simulink model "zeroovershoot"  (R2023a)
settings: Solver=VariableStepAuto  StartTime=0.0  StopTime=30  RelTol=1e-3
model workspace (MAT data in the model file):
  lambda = 0.98
libraries: slpidlib x2, cstblocks x1
settings Model: Creator=ritwi  LastModifiedBy=ritwi

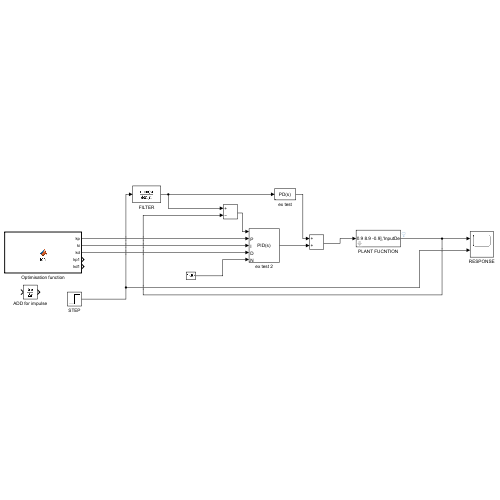
[thumbnail: Simulink's stored preview of the top-level diagram]
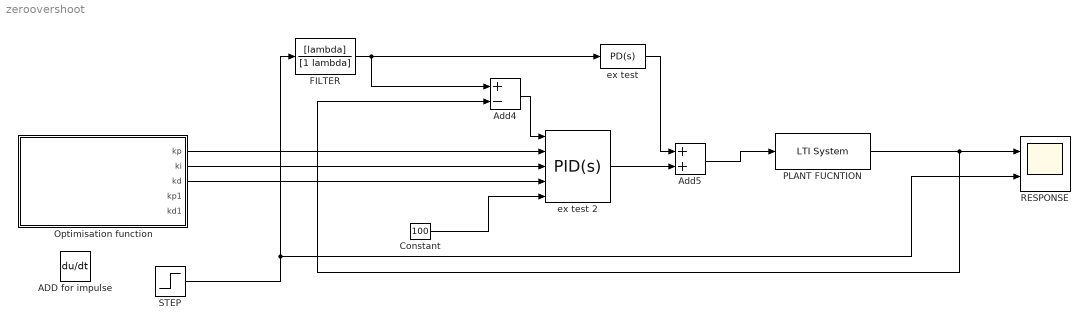
== system zeroovershoot ==
  ADD for impulse : Derivative
  Add4 : Sum  Inputs=+-
  Add5 : Sum
  Constant : Constant  Value=100
  FILTER : TransferFcn  Numerator=[lambda]  Denominator=[1 lambda]
  Optimisation function : MATLAB Function  TreatAsAtomicUnit=on
  PLANT FUCNTION : cstblocks/LTI System  sys=tf([1 ],[1 0.9 8.9 -0.9],'InputDelay',0.2)  IC=[]
  RESPONSE : Scope  NumInputPorts=2
  STEP : Step  After=1000  SampleTime=0
  ex test : slpidlib/PID Controller  Controller=PD  Form=Parallel  TimeDomain=Continuous-time  UseExternalTs=off  SampleTime=-1  IntegratorMethod=Forward Euler  FilterMethod=Forward Euler  ControllerParametersSource=internal  P=-1.2562  I=0  UseKiTs=off  D=7.6042  N=1000  UseFilter=on  TunerSelectOption=Transfer Function Based (PID Tuner App)  InitialConditionSource=internal  InitialConditionForIntegrator=0  InitialConditionForFilter=0  DifferentiatorICPrevScaledInput=0  ExternalReset=none  TrackingMode=off  Kt=1  LimitOutput=off  SatLimitsSource=internal  UpperSaturationLimit=inf  LowerSaturationLimit=-inf  LinearizeAsGain=on  AntiWindupMode=none  Kb=1  LimitIntegrator=off  UpperIntegratorSaturationLimit=inf  LowerIntegratorSaturationLimit=-inf  POutMin=[]  POutMax=[]  IOutMin=[]  IOutMax=[]  DOutMin=[]  DOutMax=[]  NOutMin=[]  NOutMax=[]  SumOutMin=[]  SumOutMax=[]  SaturationOutMin=[]  SaturationOutMax=[]  PParamMin=[]  PParamMax=[]  IParamMin=[]  IParamMax=[]  DParamMin=[]  DParamMax=[]  NParamMin=[]  NParamMax=[]  KbParamMin=[]  KbParamMax=[]  KtParamMin=[]  KtParamMax=[]  KbOutMin=[]  KbOutMax=[]  KtOutMin=[]  KtOutMax=[]  IntegratorOutMin=[]  IntegratorOutMax=[]  FilterOutMin=[]  FilterOutMax=[]  SumI1OutMin=[]  SumI1OutMax=[]  SumI2OutMin=[]  SumI2OutMax=[]  SumI3OutMin=[]  SumI3OutMax=[]  SumI4OutMin=[]  SumI4OutMax=[]  SumDOutMin=[]  SumDOutMax=[]  DifferentiatorOutMin=[]  DifferentiatorOutMax=[]  FilterDiffOutCoefMin=[]  FilterDiffOutCoefMax=[]  ReciprocalOutMin=[]  ReciprocalOutMax=[]  SumDenOutMin=[]  SumDenOutMax=[]  SumNumOutMin=[]  SumNumOutMax=[]  DivideOutMin=[]  DivideOutMax=[]  UdiffTsProdOutMin=[]  UdiffTsProdOutMax=[]  NTsProdOutMin=[]  NTsProdOutMax=[]  UintegralTsProdOutMin=[]  UintegralTsProdOutMax=[]  UngainTsProdOutMin=[]  UngainTsProdOutMax=[]  ClampingZeroOutDataTypeStr=Inherit: Inherit via back propagation  ClampingZeroOutMin=[]  ClampingZeroOutMax=[]  FilterDenConstantOutDataTypeStr=Inherit: Inherit via back propagation  FilterDenConstantOutMin=[]  FilterDenConstantOutMax=[]  PCopyOutDataTypeStr=Inherit: Inherit via back propagation  PCopyOutMin=[]  PCopyOutMax=[]  NCopyOutDataTypeStr=Inherit: Inherit via back propagation  NCopyOutMin=[]  NCopyOutMax=[]  IntegratorContinuousStateAttributes=''  IntegratorStateMustResolveToSignalObject=off  IntegratorRTWStateStorageClass=Auto  FilterContinuousStateAttributes=''  FilterStateMustResolveToSignalObject=off  FilterRTWStateStorageClass=Auto  ParallelPVariant=InternalParameters  IdealPVariant=Disabled  IVariant=Disabled  DVariant=InternalParameters  IntegratorVariant=Disabled  SatVariant=Disabled  AWVariant=Disabled  PCopyVariant=Disabled  TRVariant=Disabled  FdbkBlocksVariant=Forward  IdealPFdbkVariant=Disabled  SatFdbkVariant=Disabled  DerivativeFilterVariant=ContFilter  NVariant=InternalParameters  NCopyVariant=Disabled  FilterICVariant=InternalICsFilter  IntegratorICVariant=Disabled  ExternalResetVariant=Disabled  TRSumVariant=Passthrough  SumFdbkVariant=Disabled  SumVariant=Sum_PD  TsampFilterVariant=InternalTs  TsampNgainVariant=Passthrough  TsampIntegralVariant=Disabled_SignalSpec  ExternalSaturationOutDataTypeStr=Inherit: Same as second input
  ex test 2 : slpidlib/PID Controller  Controller=PID  Form=Parallel  TimeDomain=Continuous-time  UseExternalTs=off  SampleTime=-1  IntegratorMethod=Forward Euler  FilterMethod=Forward Euler  ControllerParametersSource=external  P=2  I=0.2942  UseKiTs=off  D=-5.8861  N=100  UseFilter=on  TunerSelectOption=Transfer Function Based (PID Tuner App)  InitialConditionSource=internal  InitialConditionForIntegrator=0  InitialConditionForFilter=0  DifferentiatorICPrevScaledInput=0  ExternalReset=none  TrackingMode=off  Kt=1  LimitOutput=off  SatLimitsSource=internal  UpperSaturationLimit=inf  LowerSaturationLimit=-inf  LinearizeAsGain=on  AntiWindupMode=none  Kb=1  LimitIntegrator=off  UpperIntegratorSaturationLimit=inf  LowerIntegratorSaturationLimit=-inf  POutMin=[]  POutMax=[]  IOutMin=[]  IOutMax=[]  DOutMin=[]  DOutMax=[]  NOutMin=[]  NOutMax=[]  SumOutMin=[]  SumOutMax=[]  SaturationOutMin=[]  SaturationOutMax=[]  PParamMin=[]  PParamMax=[]  IParamMin=[]  IParamMax=[]  DParamMin=[]  DParamMax=[]  NParamMin=[]  NParamMax=[]  KbParamMin=[]  KbParamMax=[]  KtParamMin=[]  KtParamMax=[]  KbOutMin=[]  KbOutMax=[]  KtOutMin=[]  KtOutMax=[]  IntegratorOutMin=[]  IntegratorOutMax=[]  FilterOutMin=[]  FilterOutMax=[]  SumI1OutMin=[]  SumI1OutMax=[]  SumI2OutMin=[]  SumI2OutMax=[]  SumI3OutMin=[]  SumI3OutMax=[]  SumI4OutMin=[]  SumI4OutMax=[]  SumDOutMin=[]  SumDOutMax=[]  DifferentiatorOutMin=[]  DifferentiatorOutMax=[]  FilterDiffOutCoefMin=[]  FilterDiffOutCoefMax=[]  ReciprocalOutMin=[]  ReciprocalOutMax=[]  SumDenOutMin=[]  SumDenOutMax=[]  SumNumOutMin=[]  SumNumOutMax=[]  DivideOutMin=[]  DivideOutMax=[]  UdiffTsProdOutMin=[]  UdiffTsProdOutMax=[]  NTsProdOutMin=[]  NTsProdOutMax=[]  UintegralTsProdOutMin=[]  UintegralTsProdOutMax=[]  UngainTsProdOutMin=[]  UngainTsProdOutMax=[]  ClampingZeroOutDataTypeStr=Inherit: Inherit via back propagation  ClampingZeroOutMin=[]  ClampingZeroOutMax=[]  FilterDenConstantOutDataTypeStr=Inherit: Inherit via back propagation  FilterDenConstantOutMin=[]  FilterDenConstantOutMax=[]  PCopyOutDataTypeStr=Inherit: Inherit via back propagation  PCopyOutMin=[]  PCopyOutMax=[]  NCopyOutDataTypeStr=Inherit: Inherit via back propagation  NCopyOutMin=[]  NCopyOutMax=[]  IntegratorContinuousStateAttributes=''  IntegratorStateMustResolveToSignalObject=off  IntegratorRTWStateStorageClass=Auto  FilterContinuousStateAttributes=''  FilterStateMustResolveToSignalObject=off  FilterRTWStateStorageClass=Auto  ParallelPVariant=ExternalParameters  IdealPVariant=Disabled  IVariant=ExternalParameters  DVariant=ExternalParameters  IntegratorVariant=Continuous  SatVariant=Disabled  AWVariant=Passthrough  PCopyVariant=Disabled  TRVariant=Disabled  FdbkBlocksVariant=Forward  IdealPFdbkVariant=Disabled  SatFdbkVariant=Disabled  DerivativeFilterVariant=ContFilter  NVariant=ExternalParameters  NCopyVariant=Disabled  FilterICVariant=InternalICsFilter  IntegratorICVariant=InternalICs  ExternalResetVariant=Disabled  TRSumVariant=Passthrough  SumFdbkVariant=Disabled  SumVariant=Sum_PID  TsampFilterVariant=InternalTs  TsampNgainVariant=Passthrough  TsampIntegralVariant=Disabled_SignalSpec  ExternalSaturationOutDataTypeStr=Inherit: Same as second input
  wires:
  Optimisation function/1(kp) -> ex test 2/2
  ex test 2/1 -> Add5/2
  FILTER/1 -> Add4/1, ex test/1
  ex test/1 -> Add5/1
  PLANT FUCNTION/1 -> Add4/2, RESPONSE/1
  Add4/1 -> ex test 2/1
  Add5/1 -> PLANT FUCNTION/1
  Constant/1 -> ex test 2/5
  Optimisation function/2(ki) -> ex test 2/3
  Optimisation function/3(kd) -> ex test 2/4
  STEP/1 -> FILTER/1, RESPONSE/2

== matlab function zeroovershoot/Optimisation function ==
  data: kp output; ki output; kd output; kp1 output; kd1 output
function [kp,ki, kd,kp1,kd1] = fcn
    alpha=1;
    beta=1;
    kp=2;
    A=1/(2*alpha).*real(-1./gpoletest(-1*alpha+beta*1i))+1/(2*beta).*imag(-1./gpoletest(-1*alpha+beta*1i));
    B=-1/(2*alpha).*real(-1./gpoletest(-1*alpha+beta*1i))+1/(2*beta).*imag(-1./gpoletest(-1*alpha+beta*1i));
    ki=(alpha^2+beta^2)/(2*alpha)*kp-(alpha^2+beta^2)*A;
    kd=1/(2*alpha)*kp+B;
    e=exp(1);
    func=@(s) (1).*exp(-.2.*s).*(kd.*s.^2+kp.*s+ki)+ s.*(s-0.1).*(s.^2+s+9);
    A11_=@(s) s.*(s.^2+2.*alpha.*s+alpha^2+beta^2)./func(s);
    A12_=@(s) (s.^2+2.*alpha.*s+alpha^2+beta^2)./func(s);
    B1_=@(s) -s.^2.*(s.^2+2*alpha.*s+alpha^2+beta^2)./func(s);
    C = [-11+5*1i -11-5*1i -5*1i 5*1i];
    A11 = integral(A11_,1,1,'Waypoints',C);
    A12 = integral(A12_,1,1,'Waypoints',C);
    B1 = integral(B1_,1,1,'Waypoints',C);
    x0=-5;
    A21_=@(s) s.^2.*(s.^2+2.*alpha.*s+alpha^2+beta^2)./(func(s).*(s-x0));
    A22_=@(s) s.*(s.^2+2.*alpha.*s+alpha^2+beta^2)./(func(s).*(s-x0));
    B2_=@(s) -s.^3.*(s.^2+2*alpha.*s+alpha^2+beta^2)./(func(s).*(s-x0));
    A21 = integral(A21_,1,1,'Waypoints',C);
    A22 = integral(A22_,1,1,'Waypoints',C);
    B2 = integral(B2_,1,1,'Waypoints',C);
    Amat=[A11 A12;A21 A22];
    Bmat=[B1;B2];
    Xmat=(Amat\Bmat);
    kp1=real(-ki*(Xmat(1))/Xmat(2)-kp);
    
    kd1=real(ki/Xmat(2)-kd);
    function y=gpoletest(s)
        y=1.*exp(-.2*s)/((s^2+s+9).*(s-.1));
    end
end
